simulink model "AGMD_model_R2024b"  (R2024b)
settings: Solver=VariableStepAuto  StartTime=0.0  StopTime=10.0  RelTol=1e-3
settings Model: Creator=Jan.Seemann  LastModifiedBy=Jan.Seemann

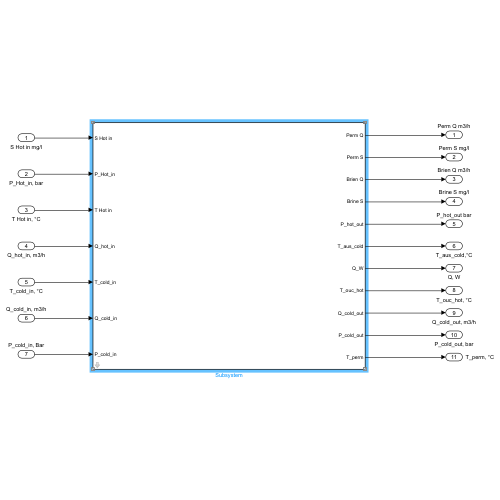
[thumbnail: Simulink's stored preview of the top-level diagram]
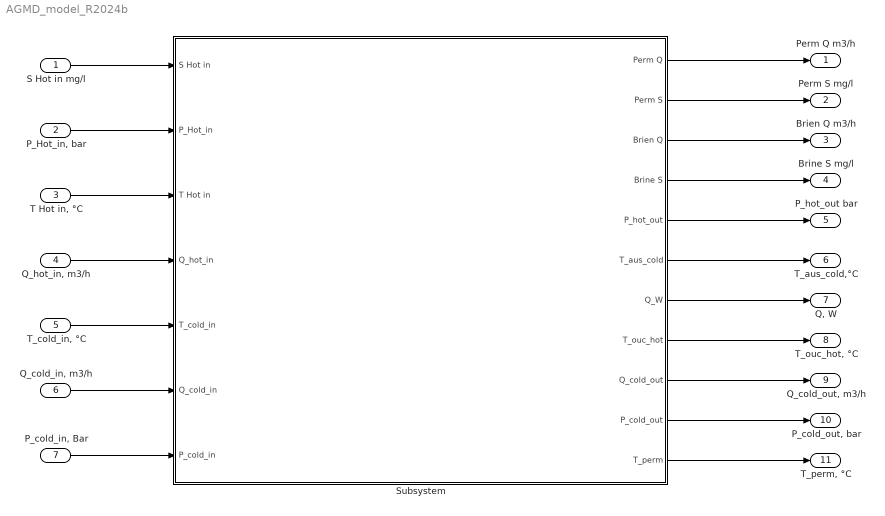
== system AGMD_model_R2024b ==
  S Hot in mg/l : Inport
  "P_Hot_in, bar" : Inport  Port=2
  "T Hot in, °C" : Inport  Port=3
  "Q_hot_in, m3/h" : Inport  Port=4
  "T_cold_in, °C" : Inport  Port=5
  "Q_cold_in, m3/h" : Inport  Port=6
  "P_cold_in, Bar" : Inport  Port=7
  Subsystem : Subsystem  mask{A=15, R=0.9999999, CCP=4000, HCP=4000, Dicke_Air=62/1000/1000, Dicke_cp=62/1000/1000, Dicke_M=69/1000/1000, K_air=0.0025, K_cp=0.5, K_m=0.25, DPCold=0, DPHOt=0, L=11.6}
      mask prompts: A "Area"; R "Recejectionratio"; CCP "heat capacity Cold Fluid, J/kgK"; HCP "heat capacity Hot Fluid, J/kgK"; Dicke_Air "Space Air, m"; Dicke_cp "thickness Cooling Platte, m"; Dicke_M "thickness Membrane, m"; K_air "Thermal conductivity Air, W/mK"; K_cp "Thermal conductivity Cooling Platte, W/mK"; K_m "Thermal conductivity Membrane, W/mK"; DPCold "Pressure drop ColdTube, bar"; DPHOt "Pressure drop Hot Tube, bar"; L "Chara. Length, m"
  Perm Q m3/h : Outport
  Perm S mg/l : Outport  Port=2
  Brien Q m3/h : Outport  Port=3
  Brine S mg/l : Outport  Port=4
  P_hot_out bar : Outport  Port=5
  T_aus_cold,°C : Outport  Port=6
  "Q, W" : Outport  Port=7
  "T_ouc_hot, °C" : Outport  Port=8
  "Q_cold_out, m3/h" : Outport  Port=9
  "P_cold_out, bar" : Outport  Port=10
  "T_perm, °C" : Outport  Port=11
  wires:
  Subsystem/1(Perm Q) -> Perm Q m3/h/1
  Subsystem/2(Perm S) -> Perm S mg/l/1
  Subsystem/3(Brien Q) -> Brien Q m3/h/1
  Subsystem/4(Brine S) -> Brine S mg/l/1
  Subsystem/5(P_hot_out) -> P_hot_out bar/1
  Subsystem/6(T_aus_cold) -> T_aus_cold,°C/1
  Subsystem/7(Q_W) -> "Q, W"/1
  Subsystem/8(T_ouc_hot) -> "T_ouc_hot, °C"/1
  Subsystem/9(Q_cold_out) -> "Q_cold_out, m3/h"/1
  Subsystem/10(P_cold_out) -> "P_cold_out, bar"/1
  Subsystem/11(T_perm) -> "T_perm, °C"/1
  S Hot in mg/l/1 -> Subsystem/1(S Hot in)
  "P_Hot_in, bar"/1 -> Subsystem/2(P_Hot_in)
  "T Hot in, °C"/1 -> Subsystem/3(T Hot in)
  "Q_hot_in, m3/h"/1 -> Subsystem/4(Q_hot_in)
  "T_cold_in, °C"/1 -> Subsystem/5(T_cold_in)
  "Q_cold_in, m3/h"/1 -> Subsystem/6(Q_cold_in)
  "P_cold_in, Bar"/1 -> Subsystem/7(P_cold_in)

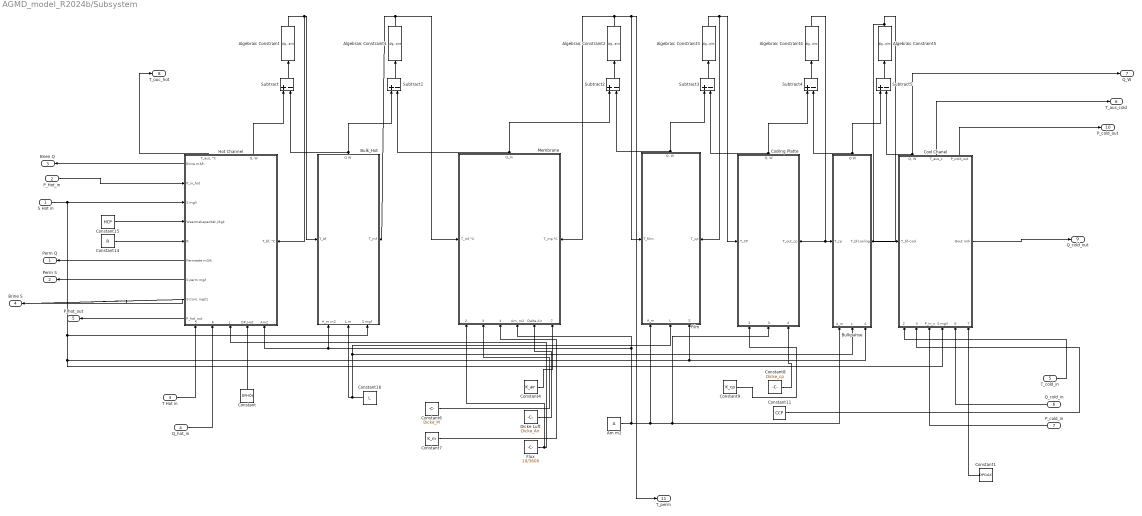
== system AGMD_model_R2024b/Subsystem ==
  S Hot in : Inport
  P_Hot_in : Inport  Port=2
  T Hot in : Inport  Port=3
  Q_hot_in : Inport  Port=4
  T_cold_in : Inport  Port=5
  Q_cold_in : Inport  Port=6
  P_cold_in : Inport  Port=7
  Algebraic Constraint{,1..5} (6 alike) : AlgebraicConstraint
  Am m2 : Constant  Value=A
  Bulk_Hot : Subsystem
      settings: PortSchema="{\"entries\":[{\"content\":{\"sides\":[{\"content\":{\"connectorIds\":[\"In1\"]},\"type\":\"ConnectorPlacement.EquallySpacedRectSide\",\"uuid\":\"ef4b2b41-cf19-4205-8bdd-c88c0c8e6088\"},{\"content\":{\"connectorIds\":[\"In5\"],\"side\":\"RIGHT\"},\"type\":\"ConnectorPlacement.EquallySpacedRectSide\",\"uuid\":\"90a0e595-a90d-4955-971b-cbb17d54f339\"},{\"content\":{\"connectorIds\":[\"Out1\"],\"side\":\"TOP\"},\"type\":\"ConnectorPlacement.EquallySpacedRectSide\",\"uuid\":\"ac71d737-c091-4b4d-923a-bfea117e1c9e\"},{\"content\":{\"connectorIds\":[\"In2\",\"In3\",\"In4\"],\"side\":\"BOTTOM\"},\"type\":\"ConnectorPlacement.EquallySpacedRectSide\",\"uuid\":\"c078efbb-00a2-4bad-921f-0a538f18104b\"}]},\"type\":\"ConnectorPlacement.EquallySpacedConnector\",\"uuid\":\"3aaa503e-a2b4-481c-8e52-42dcdd859844\"}],\"packageUris\":[\"http://schema.mathworks.com/mf0/Connector/R2020b\"],\"version\":\"1.0\"}"
  Bulkpahse : Subsystem
      settings: PortSchema="{\"entries\":[{\"content\":{\"sides\":[{\"content\":{\"connectorIds\":[\"In1\"]},\"type\":\"ConnectorPlacement.EquallySpacedRectSide\",\"uuid\":\"cd83c780-39a7-488d-a3d5-66e3425d7f86\"},{\"content\":{\"connectorIds\":[\"In5\"],\"side\":\"RIGHT\"},\"type\":\"ConnectorPlacement.EquallySpacedRectSide\",\"uuid\":\"ad4f5b7f-34f2-414c-8bc1-990d5ddf120f\"},{\"content\":{\"connectorIds\":[\"Out1\"],\"side\":\"TOP\"},\"type\":\"ConnectorPlacement.EquallySpacedRectSide\",\"uuid\":\"d94043ec-1d76-4835-9fe5-55fe607ca13f\"},{\"content\":{\"connectorIds\":[\"In2\",\"In3\",\"In4\"],\"side\":\"BOTTOM\"},\"type\":\"ConnectorPlacement.EquallySpacedRectSide\",\"uuid\":\"b1fdfa3b-d721-4849-9383-0fd7a2ff7ce1\"}]},\"type\":\"ConnectorPlacement.EquallySpacedConnector\",\"uuid\":\"49b2ce75-7c12-4465-a9d1-22146559eb16\"}],\"packageUris\":[\"http://schema.mathworks.com/mf0/Connector/R2020b\"],\"version\":\"1.0\"}"
  Constant : Constant  Value=DPHOt
  Constant1 : Constant  Value=DPCold
  Constant11 : Constant  Value=CCP
  Constant14 : Constant  Value=R
  Constant15 : Constant  Value=HCP
  Constant16 : Constant  Value=L
  Constant4 : Constant  Value=K_air
  Constant6 : Constant  Value=Dicke_M
  Constant7 : Constant  Value=K_m
  Constant8 : Constant  Value=Dicke_cp
  Constant9 : Constant  Value=K_cp
  Cool Chanel : Subsystem
      settings: PortSchema="{\"entries\":[{\"content\":{\"sides\":[{\"content\":{\"connectorIds\":[\"In1\"]},\"type\":\"ConnectorPlacement.EquallySpacedRectSide\",\"uuid\":\"c448acfc-f6aa-48b6-b853-5d81d9281dc0\"},{\"content\":{\"connectorIds\":[\"Out1\"],\"side\":\"RIGHT\"},\"type\":\"ConnectorPlacement.EquallySpacedRectSide\",\"uuid\":\"7e575c83-2c86-4510-ae36-745e6aa83247\"},{\"content\":{\"connectorIds\":[\"Out2\",\"Out3\",\"Out4\"],\"side\":\"TOP\"},\"type\":\"ConnectorPlacement.EquallySpacedRectSide\",\"uuid\":\"4a6df9d2-b5c9-43f7-a3d9-0ac9bbe4b67a\"},{\"content\":{\"connectorIds\":[\"In2\",\"In3\",\"In4\",\"In5\",\"In6\",\"In7\"],\"side\":\"BOTTOM\"},\"type\":\"ConnectorPlacement.EquallySpacedRectSide\",\"uuid\":\"eac96ba6-fa95-4e63-96f7-b902511d10a6\"}]},\"type\":\"ConnectorPlacement.EquallySpacedConnector\",\"uuid\":\"289f5ba6-df51-43a8-9e65-4dc3058f2d7c\"}],\"packageUris\":[\"http://schema.mathworks.com/mf0/Connector/R2020b\"],\"version\":\"1.0\"}"
  Cooling Platte : Subsystem
      settings: PortSchema="{\"entries\":[{\"content\":{\"sides\":[{\"content\":{\"connectorIds\":[\"In1\"]},\"type\":\"ConnectorPlacement.EquallySpacedRectSide\",\"uuid\":\"c07f3d14-23da-4d6c-a231-b487d35cf23a\"},{\"content\":{\"connectorIds\":[\"In5\"],\"side\":\"RIGHT\"},\"type\":\"ConnectorPlacement.EquallySpacedRectSide\",\"uuid\":\"132dff7f-1270-4e73-a49f-8e3c493cbf76\"},{\"content\":{\"connectorIds\":[\"Out1\"],\"side\":\"TOP\"},\"type\":\"ConnectorPlacement.EquallySpacedRectSide\",\"uuid\":\"f42b61b3-9665-4b68-99ce-b4151b983a04\"},{\"content\":{\"connectorIds\":[\"In2\",\"In3\",\"In4\"],\"side\":\"BOTTOM\"},\"type\":\"ConnectorPlacement.EquallySpacedRectSide\",\"uuid\":\"3d6787e6-2f20-4c5d-b35a-cc189669d767\"}]},\"type\":\"ConnectorPlacement.EquallySpacedConnector\",\"uuid\":\"48e32856-75ee-4ce0-8b78-4952240158a6\"}],\"packageUris\":[\"http://schema.mathworks.com/mf0/Connector/R2020b\"],\"version\":\"1.0\"}"
  "Dicke Luft " : Constant  Value=Dicke_Air
  Film : Subsystem
      settings: PortSchema="{\"entries\":[{\"content\":{\"sides\":[{\"content\":{\"connectorIds\":[\"In1\"]},\"type\":\"ConnectorPlacement.EquallySpacedRectSide\",\"uuid\":\"015337e1-8a5a-4833-8b0f-5ab9d6f3a80e\"},{\"content\":{\"connectorIds\":[\"In5\"],\"side\":\"RIGHT\"},\"type\":\"ConnectorPlacement.EquallySpacedRectSide\",\"uuid\":\"ffe29c11-abce-4f62-86d7-78803d541e75\"},{\"content\":{\"connectorIds\":[\"Out1\"],\"side\":\"TOP\"},\"type\":\"ConnectorPlacement.EquallySpacedRectSide\",\"uuid\":\"6e7e379e-b700-4f80-905d-b6d3887cb320\"},{\"content\":{\"connectorIds\":[\"In2\",\"In3\",\"In4\"],\"side\":\"BOTTOM\"},\"type\":\"ConnectorPlacement.EquallySpacedRectSide\",\"uuid\":\"39f7c5ec-6303-4d87-b419-58dfdd6ec091\"}]},\"type\":\"ConnectorPlacement.EquallySpacedConnector\",\"uuid\":\"e7928b9b-306f-421e-9818-1e4095991db6\"}],\"packageUris\":[\"http://schema.mathworks.com/mf0/Connector/R2020b\"],\"version\":\"1.0\"}"
  Flux : Constant  Value=10/3600
  Hot Channel : Subsystem
      settings: PortSchema="{\"entries\":[{\"content\":{\"sides\":[{\"content\":{\"connectorIds\":[\"Out3\",\"In1\",\"In2\",\"In3\",\"In4\",\"Out4\",\"Out5\",\"Out6\",\"Out7\"]},\"type\":\"ConnectorPlacement.EquallySpacedRectSide\",\"uuid\":\"fbc7a68d-5beb-43dd-a6f0-b755d0c17893\"},{\"content\":{\"connectorIds\":[\"In10\"],\"side\":\"RIGHT\"},\"type\":\"ConnectorPlacement.EquallySpacedRectSide\",\"uuid\":\"0716d393-5c1b-482d-88d7-1d54bbed30c8\"},{\"content\":{\"connectorIds\":[\"Out1\",\"Out2\"],\"side\":\"TOP\"},\"type\":\"ConnectorPlacement.EquallySpacedRectSide\",\"uuid\":\"7cadc919-8496-492b-8ec9-a6875040d21a\"},{\"content\":{\"connectorIds\":[\"In5\",\"In6\",\"In7\",\"In8\",\"In9\"],\"side\":\"BOTTOM\"},\"type\":\"ConnectorPlacement.EquallySpacedRectSide\",\"uuid\":\"ee11a940-0fee-47a3-9594-370a89fbc708\"}]},\"type\":\"ConnectorPlacement.EquallySpacedConnector\",\"uuid\":\"ba3bcdcd-a15a-4c6e-8936-726ab8cfa6f6\"}],\"packageUris\":[\"http://schema.mathworks.com/mf0/Connector/R2020b\"],\"version\":\"1.0\"}"
  Membrane : Subsystem
      settings: PortSchema="{\"entries\":[{\"content\":{\"sides\":[{\"content\":{\"connectorIds\":[\"In1\"]},\"type\":\"ConnectorPlacement.EquallySpacedRectSide\",\"uuid\":\"cd69aa9c-a695-4ae3-919f-da2064161930\"},{\"content\":{\"connectorIds\":[\"In8\"],\"side\":\"RIGHT\"},\"type\":\"ConnectorPlacement.EquallySpacedRectSide\",\"uuid\":\"a625c06c-887d-4646-98b1-3b4393effb73\"},{\"content\":{\"connectorIds\":[\"Out1\"],\"side\":\"TOP\"},\"type\":\"ConnectorPlacement.EquallySpacedRectSide\",\"uuid\":\"4b547f2f-723c-4068-9bd6-c942a8ec2112\"},{\"content\":{\"connectorIds\":[\"In2\",\"In3\",\"In4\",\"In5\",\"In6\",\"In7\"],\"side\":\"BOTTOM\"},\"type\":\"ConnectorPlacement.EquallySpacedRectSide\",\"uuid\":\"bf68c9ad-e157-4c0d-9a2b-c7fd1689a3f4\"}]},\"type\":\"ConnectorPlacement.EquallySpacedConnector\",\"uuid\":\"d2d78d85-b2cf-48d3-9a1a-b69a88097481\"}],\"packageUris\":[\"http://schema.mathworks.com/mf0/Connector/R2020b\"],\"version\":\"1.0\"}"
  Subtract{,1..5} (6 alike) : Sum  Inputs=+-
  Perm Q : Outport
  Perm S : Outport  Port=2
  Brien Q : Outport  Port=3
  Brine S : Outport  Port=4
  P_hot_out : Outport  Port=5
  T_aus_cold : Outport  Port=6
  Q_W : Outport  Port=7
  T_ouc_hot : Outport  Port=8
  Q_cold_out : Outport  Port=9
  P_cold_out : Outport  Port=10
  T_perm : Outport  Port=11
  wires:
  Algebraic Constraint1/1 -> Membrane/1(T_mf,°C), Bulk_Hot/5(T_mf)
  Q_hot_in/1 -> Hot Channel/6(Q Hot m3/h)
  Hot Channel/5(S perm mg/l) -> Perm S/1
  Constant8/1 -> Cooling Platte/4(Delta Paltte Cooling)
  Cool Chanel/3(T_aus_c) -> T_aus_cold/1
  Membrane/1(Q_m) -> Subtract1/2, Subtract2/1
  Constant9/1 -> Cooling Platte/2(Waermeleitfaehigkeit Platte)
  Subtract5/1 -> Algebraic Constraint5/1
  Bulk_Hot/1(Q W) -> Subtract/2, Subtract1/1
  Cool Chanel/4(P_cold_out) -> P_cold_out/1
  Am m2/1 -> Bulkpahse/2(A_m), Cooling Platte/3(Flaeche der Cooling Platte), Film/2(A_m), Hot Channel/9(Am2), Bulk_Hot/2(A_m m2), Membrane/5("Am, m2")
  Constant11/1 -> Cool Chanel/3(Waermekapazität J/kgK)
  Subtract1/1 -> Algebraic Constraint1/1
  Cool Chanel/1(Qout m/h) -> Q_cold_out/1
  S Hot in/1 -> Bulkpahse/4(S), Film/4(S), Cool Chanel/5(S mg/l), Bulk_Hot/4(S mg/l), Hot Channel/2(S mg/l)
  Algebraic Constraint4/1 -> Cooling Platte/5(T_out_cp), Bulkpahse/1(T_cp)
  Subtract/1 -> Algebraic Constraint/1
  Algebraic Constraint5/1 -> Cool Chanel/1(T_bf-cool), Bulkpahse/5(T_bfcooling)
  P_cold_in/1 -> Cool Chanel/4(P_in_c)
  "Dicke Luft "/1 -> Membrane/6(Dalta Air)
  T_cold_in/1 -> Cool Chanel/2(T_cooling_ein)
  P_Hot_in/1 -> Hot Channel/1(P_in_hot)
  Cool Chanel/2("Q, W") -> Q_W/1, Subtract5/2
  Constant16/1 -> Bulkpahse/3(L), Film/3(L), Bulk_Hot/3(L m)
  Hot Channel/1("T_aus, °C") -> T_ouc_hot/1
  Bulkpahse/1(Q W) -> Subtract5/1, Subtract4/2
  Hot Channel/7(P_hot_out) -> P_hot_out/1
  Hot Channel/6(S Conc mg/l1) -> Brine S/1
  Flux/1 -> Hot Channel/7(J), Membrane/2("J, kg/sm2")
  Constant14/1 -> Hot Channel/4(R)
  Film/1("Q, W") -> Subtract2/2, Subtract3/1
  Subtract3/1 -> Algebraic Constraint3/1
  T Hot in/1 -> Hot Channel/5("T_h_ein, °C")
  Q_cold_in/1 -> Cool Chanel/6(Q cold m3/h)
  Constant4/1 -> Membrane/7("k_air, W/mK")
  Hot Channel/3(Brine m3/h) -> Brien Q/1
  Constant1/1 -> Cool Chanel/7(DPCOld)
  Algebraic Constraint3/1 -> Cooling Platte/1(T_CP), Film/5(T_cp)
  Constant15/1 -> Hot Channel/3(Waermekapazität j/kgk)
  Algebraic Constraint2/1 -> T_perm/1, Film/1(T_film), Membrane/8(T_mp,°C)
  Subtract4/1 -> Algebraic Constraint4/1
  Constant7/1 -> Membrane/4("k_m, W/mK")
  Constant6/1 -> Membrane/3("delta_m, m")
  Hot Channel/4(Permeate m3/h) -> Perm Q/1
  Constant/1 -> Hot Channel/8(DP_Hot)
  Cooling Platte/1("Q, W") -> Subtract3/2, Subtract4/1
  Algebraic Constraint/1 -> Hot Channel/10("T_bf, °C"), Bulk_Hot/1(T_bf)
  Hot Channel/2("Q, W") -> Subtract/1
  Subtract2/1 -> Algebraic Constraint2/1

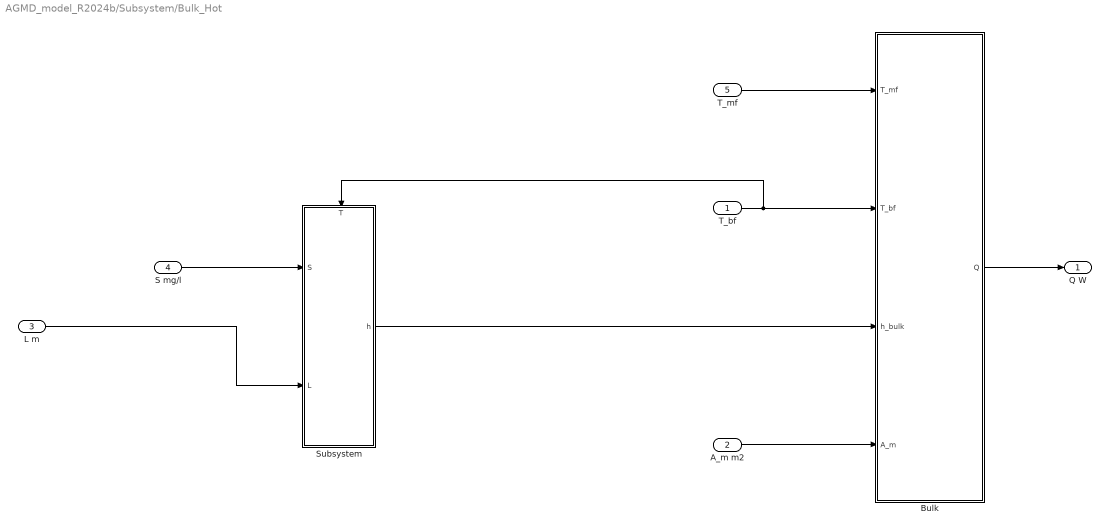
== system AGMD_model_R2024b/Subsystem/Bulk_Hot ==
  T_bf : Inport
  A_m m2 : Inport  Port=2
  L m : Inport  Port=3
  S mg/l : Inport  Port=4
  T_mf : Inport  Port=5
  Bulk : MATLAB Function  TreatAsAtomicUnit=on
  Subsystem : Subsystem
      settings: PortSchema="{\"entries\":[{\"content\":{\"sides\":[{\"content\":{\"connectorIds\":[\"In1\",\"In2\"]},\"type\":\"ConnectorPlacement.EquallySpacedRectSide\",\"uuid\":\"4135ebe6-441f-43d7-9be9-d9525d176f2c\"},{\"content\":{\"connectorIds\":[\"Out1\"],\"side\":\"RIGHT\"},\"type\":\"ConnectorPlacement.EquallySpacedRectSide\",\"uuid\":\"d9e7871b-5841-4db7-96fe-8558ee3ebd7a\"},{\"content\":{\"connectorIds\":[\"In3\"],\"side\":\"TOP\"},\"type\":\"ConnectorPlacement.EquallySpacedRectSide\",\"uuid\":\"bca1fa39-ae4b-46e6-af8d-7fe20692a0ee\"}]},\"type\":\"ConnectorPlacement.EquallySpacedConnector\",\"uuid\":\"33afa6da-10b0-4c15-8b5e-951d2ae663b7\"}],\"packageUris\":[\"http://schema.mathworks.com/mf0/Connector/R2020b\"],\"version\":\"1.0\"}"
  Q W : Outport
  wires:
  Bulk/1(Q) -> Q W/1
  T_mf/1 -> Bulk/1(T_mf)
  T_bf/1 -> Bulk/2(T_bf), Subsystem/3(T)
  A_m m2/1 -> Bulk/4(A_m)
  S mg/l/1 -> Subsystem/1(S)
  L m/1 -> Subsystem/2(L)
  Subsystem/1(h) -> Bulk/3(h_bulk)

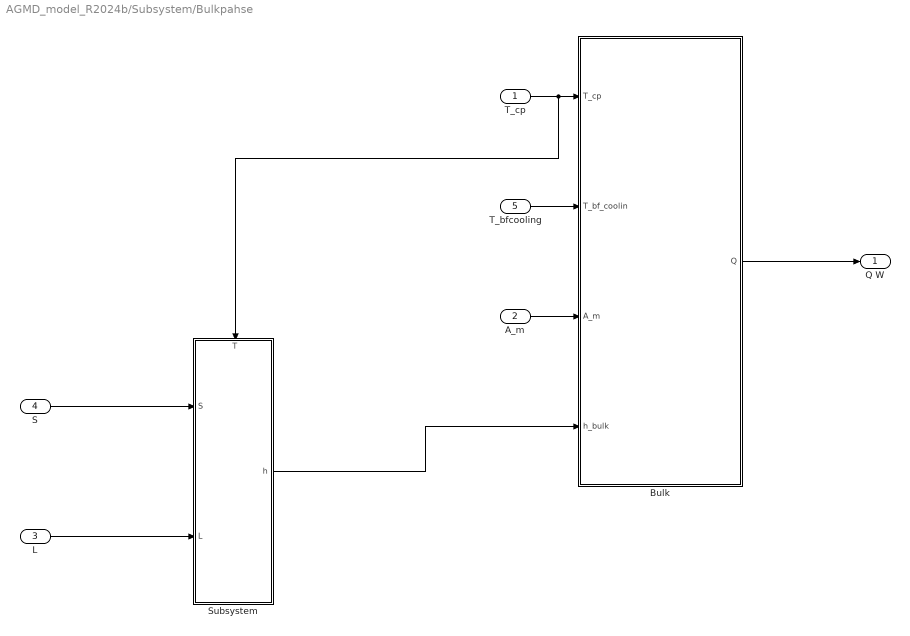
== system AGMD_model_R2024b/Subsystem/Bulkpahse ==
  T_cp : Inport
  A_m : Inport  Port=2
  L : Inport  Port=3
  S : Inport  Port=4
  T_bfcooling : Inport  Port=5
  Bulk : MATLAB Function  TreatAsAtomicUnit=on
  Subsystem : Subsystem
      settings: PortSchema="{\"entries\":[{\"content\":{\"sides\":[{\"content\":{\"connectorIds\":[\"In1\",\"In2\"]},\"type\":\"ConnectorPlacement.EquallySpacedRectSide\",\"uuid\":\"4135ebe6-441f-43d7-9be9-d9525d176f2c\"},{\"content\":{\"connectorIds\":[\"Out1\"],\"side\":\"RIGHT\"},\"type\":\"ConnectorPlacement.EquallySpacedRectSide\",\"uuid\":\"d9e7871b-5841-4db7-96fe-8558ee3ebd7a\"},{\"content\":{\"connectorIds\":[\"In3\"],\"side\":\"TOP\"},\"type\":\"ConnectorPlacement.EquallySpacedRectSide\",\"uuid\":\"bca1fa39-ae4b-46e6-af8d-7fe20692a0ee\"}]},\"type\":\"ConnectorPlacement.EquallySpacedConnector\",\"uuid\":\"33afa6da-10b0-4c15-8b5e-951d2ae663b7\"}],\"packageUris\":[\"http://schema.mathworks.com/mf0/Connector/R2020b\"],\"version\":\"1.0\"}"
  Q W : Outport
  wires:
  Bulk/1(Q) -> Q W/1
  T_cp/1 -> Subsystem/3(T), Bulk/1(T_cp)
  T_bfcooling/1 -> Bulk/2(T_bf_coolin)
  A_m/1 -> Bulk/3(A_m)
  S/1 -> Subsystem/1(S)
  L/1 -> Subsystem/2(L)
  Subsystem/1(h) -> Bulk/4(h_bulk)

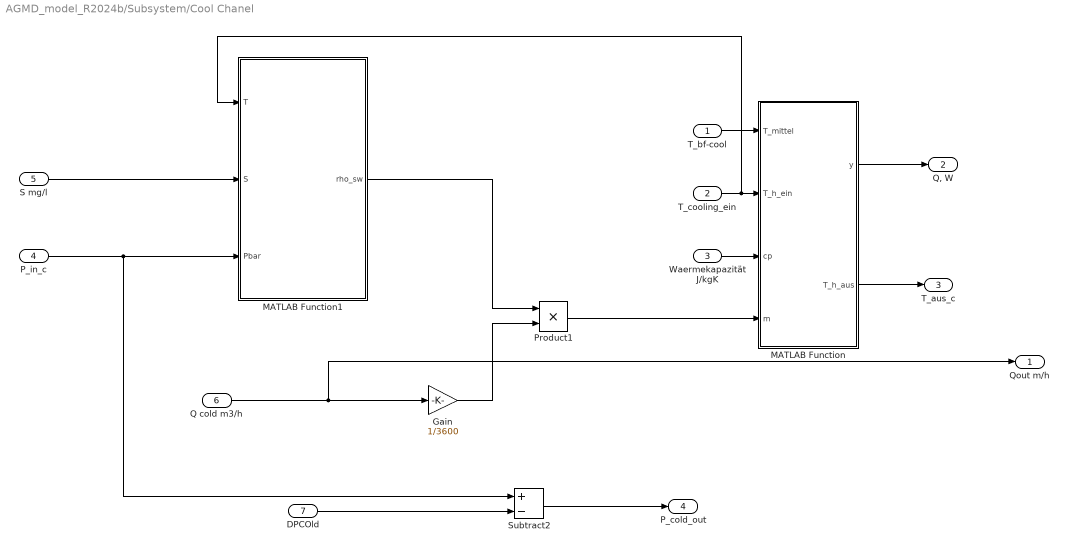
== system AGMD_model_R2024b/Subsystem/Cool Chanel ==
  T_bf-cool : Inport
  T_cooling_ein : Inport  Port=2
  Waermekapazität J/kgK : Inport  Port=3
  P_in_c : Inport  Port=4
  S mg/l : Inport  Port=5
  Q cold m3/h : Inport  Port=6
  DPCOld : Inport  Port=7
  Gain : Gain  Gain=1/3600
  MATLAB Function : MATLAB Function  TreatAsAtomicUnit=on
  MATLAB Function1 : MATLAB Function  TreatAsAtomicUnit=on
  Product1 : Product
  Subtract2 : Sum  Inputs=+-
  Qout m/h : Outport
  "Q, W" : Outport  Port=2
  T_aus_c : Outport  Port=3
  P_cold_out : Outport  Port=4
  wires:
  MATLAB Function/2(T_h_aus) -> T_aus_c/1
  MATLAB Function/1(y) -> "Q, W"/1
  T_bf-cool/1 -> MATLAB Function/1(T_mittel)
  Waermekapazität J/kgK/1 -> MATLAB Function/3(cp)
  MATLAB Function1/1(rho_sw) -> Product1/1
  T_cooling_ein/1 -> MATLAB Function1/1(T), MATLAB Function/2(T_h_ein)
  S mg/l/1 -> MATLAB Function1/2(S)
  Q cold m3/h/1 -> Qout m/h/1, Gain/1
  Gain/1 -> Product1/2
  P_in_c/1 -> Subtract2/1, MATLAB Function1/3(Pbar)
  Product1/1 -> MATLAB Function/4(m)
  Subtract2/1 -> P_cold_out/1
  DPCOld/1 -> Subtract2/2

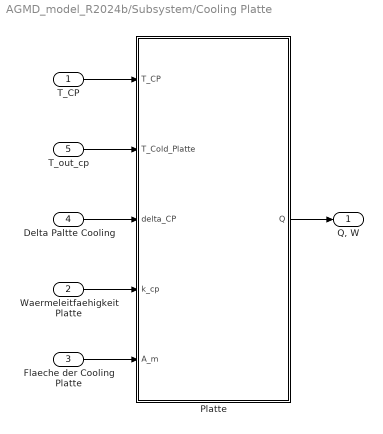
== system AGMD_model_R2024b/Subsystem/Cooling Platte ==
  T_CP : Inport
  Waermeleitfaehigkeit Platte : Inport  Port=2
  Flaeche der Cooling Platte : Inport  Port=3
  Delta Paltte Cooling : Inport  Port=4
  T_out_cp : Inport  Port=5
  Platte : MATLAB Function  TreatAsAtomicUnit=on
  "Q, W" : Outport
  wires:
  T_out_cp/1 -> Platte/2(T_Cold_Platte)
  T_CP/1 -> Platte/1(T_CP)
  Delta Paltte Cooling/1 -> Platte/3(delta_CP)
  Waermeleitfaehigkeit Platte/1 -> Platte/4(k_cp)
  Flaeche der Cooling Platte/1 -> Platte/5(A_m)
  Platte/1(Q) -> "Q, W"/1

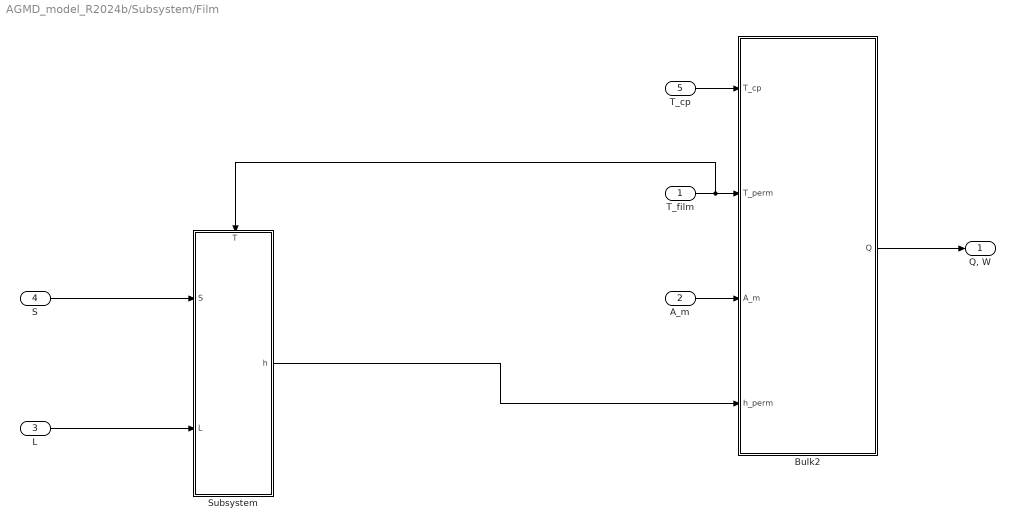
== system AGMD_model_R2024b/Subsystem/Film ==
  T_film : Inport
  A_m : Inport  Port=2
  L : Inport  Port=3
  S : Inport  Port=4
  T_cp : Inport  Port=5
  Bulk2 : MATLAB Function  TreatAsAtomicUnit=on
  Subsystem : Subsystem
      settings: PortSchema="{\"entries\":[{\"content\":{\"sides\":[{\"content\":{\"connectorIds\":[\"In1\",\"In2\"]},\"type\":\"ConnectorPlacement.EquallySpacedRectSide\",\"uuid\":\"4135ebe6-441f-43d7-9be9-d9525d176f2c\"},{\"content\":{\"connectorIds\":[\"Out1\"],\"side\":\"RIGHT\"},\"type\":\"ConnectorPlacement.EquallySpacedRectSide\",\"uuid\":\"d9e7871b-5841-4db7-96fe-8558ee3ebd7a\"},{\"content\":{\"connectorIds\":[\"In3\"],\"side\":\"TOP\"},\"type\":\"ConnectorPlacement.EquallySpacedRectSide\",\"uuid\":\"bca1fa39-ae4b-46e6-af8d-7fe20692a0ee\"}]},\"type\":\"ConnectorPlacement.EquallySpacedConnector\",\"uuid\":\"33afa6da-10b0-4c15-8b5e-951d2ae663b7\"}],\"packageUris\":[\"http://schema.mathworks.com/mf0/Connector/R2020b\"],\"version\":\"1.0\"}"
  "Q, W" : Outport
  wires:
  T_cp/1 -> Bulk2/1(T_cp)
  T_film/1 -> Subsystem/3(T), Bulk2/2(T_perm)
  Bulk2/1(Q) -> "Q, W"/1
  A_m/1 -> Bulk2/3(A_m)
  L/1 -> Subsystem/2(L)
  Subsystem/1(h) -> Bulk2/4(h_perm)
  S/1 -> Subsystem/1(S)

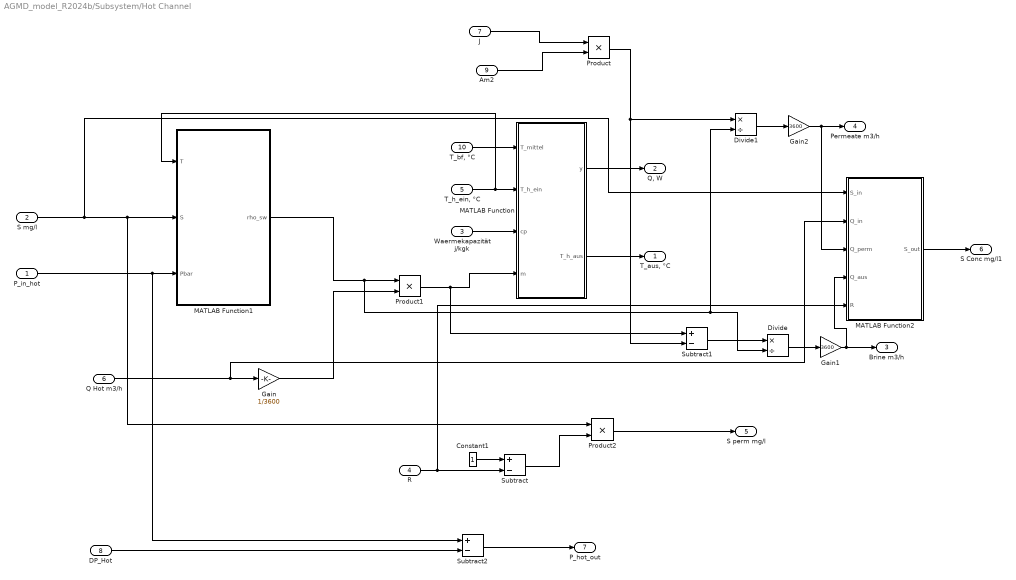
== system AGMD_model_R2024b/Subsystem/Hot Channel ==
  P_in_hot : Inport
  S mg/l : Inport  Port=2
  Waermekapazität j/kgk : Inport  Port=3
  R : Inport  Port=4
  "T_h_ein, °C" : Inport  Port=5
  Q Hot m3/h : Inport  Port=6
  J : Inport  Port=7
  DP_Hot : Inport  Port=8
  Am2 : Inport  Port=9
  "T_bf, °C" : Inport  Port=10
  Constant1 : Constant
  Divide : Product  Inputs=*/
  Divide1 : Product  Inputs=*/
  Gain : Gain  Gain=1/3600
  Gain1 : Gain  Gain=3600
  Gain2 : Gain  Gain=3600
  MATLAB Function : MATLAB Function  TreatAsAtomicUnit=on
  MATLAB Function1 : MATLAB Function  TreatAsAtomicUnit=on
  MATLAB Function2 : MATLAB Function  TreatAsAtomicUnit=on
  Product : Product
  Product1 : Product
  Product2 : Product
  Subtract : Sum  Inputs=+-
  Subtract1 : Sum  Inputs=+-
  Subtract2 : Sum  Inputs=+-
  "T_aus, °C" : Outport
  "Q, W" : Outport  Port=2
  Brine m3/h : Outport  Port=3
  Permeate m3/h : Outport  Port=4
  S perm mg/l : Outport  Port=5
  S Conc mg/l1 : Outport  Port=6
  P_hot_out : Outport  Port=7
  wires:
  J/1 -> Product/1
  MATLAB Function/1(y) -> "Q, W"/1
  "T_bf, °C"/1 -> MATLAB Function/1(T_mittel)
  Waermekapazität j/kgk/1 -> MATLAB Function/3(cp)
  MATLAB Function/2(T_h_aus) -> "T_aus, °C"/1
  "T_h_ein, °C"/1 -> MATLAB Function1/1(T), MATLAB Function/2(T_h_ein)
  R/1 -> MATLAB Function2/5(R), Subtract/2
  Constant1/1 -> Subtract/1
  Am2/1 -> Product/2
  Product/1 -> Divide1/1, Subtract1/2
  P_in_hot/1 -> Subtract2/1, MATLAB Function1/3(Pbar)
  S mg/l/1 -> MATLAB Function2/1(S_in), Product2/1, MATLAB Function1/2(S)
  Q Hot m3/h/1 -> MATLAB Function2/2(Q_in), Gain/1
  MATLAB Function1/1(rho_sw) -> Divide1/2, Divide/2, Product1/1
  Product1/1 -> Subtract1/1, MATLAB Function/4(m)
  Gain/1 -> Product1/2
  Subtract1/1 -> Divide/1
  Divide/1 -> Gain1/1
  Gain2/1 -> MATLAB Function2/3(Q_perm), Permeate m3/h/1
  Divide1/1 -> Gain2/1
  Subtract/1 -> Product2/2
  Product2/1 -> S perm mg/l/1
  MATLAB Function2/1(S_out) -> S Conc mg/l1/1
  Gain1/1 -> MATLAB Function2/4(Q_aus), Brine m3/h/1
  DP_Hot/1 -> Subtract2/2
  Subtract2/1 -> P_hot_out/1

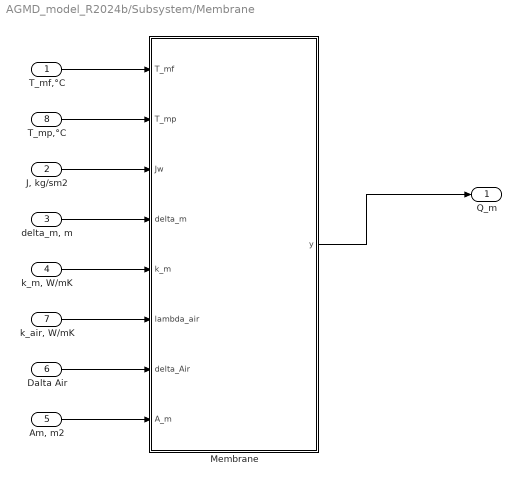
== system AGMD_model_R2024b/Subsystem/Membrane ==
  T_mf,°C : Inport
  "J, kg/sm2" : Inport  Port=2
  "delta_m, m" : Inport  Port=3
  "k_m, W/mK" : Inport  Port=4
  "Am, m2" : Inport  Port=5
  Dalta Air : Inport  Port=6
  "k_air, W/mK" : Inport  Port=7
  T_mp,°C : Inport  Port=8
  Membrane : MATLAB Function  TreatAsAtomicUnit=on
  Q_m : Outport
  wires:
  "J, kg/sm2"/1 -> Membrane/3(Jw)
  "delta_m, m"/1 -> Membrane/4(delta_m)
  "k_m, W/mK"/1 -> Membrane/5(k_m)
  "Am, m2"/1 -> Membrane/8(A_m)
  T_mf,°C/1 -> Membrane/1(T_mf)
  Membrane/1(y) -> Q_m/1
  T_mp,°C/1 -> Membrane/2(T_mp)
  "k_air, W/mK"/1 -> Membrane/6(lambda_air)
  Dalta Air/1 -> Membrane/7(delta_Air)

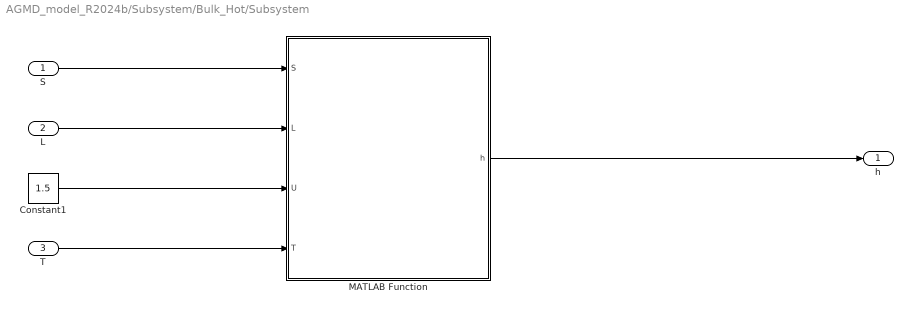
== system AGMD_model_R2024b/Subsystem/Bulk_Hot/Subsystem ==
  S : Inport
  L : Inport  Port=2
  T : Inport  Port=3
  Constant1 : Constant  Value=1.5
  MATLAB Function : MATLAB Function  TreatAsAtomicUnit=on
  h : Outport
  wires:
  L/1 -> MATLAB Function/2(L)
  MATLAB Function/1(h) -> h/1
  S/1 -> MATLAB Function/1(S)
  Constant1/1 -> MATLAB Function/3(U)
  T/1 -> MATLAB Function/4(T)

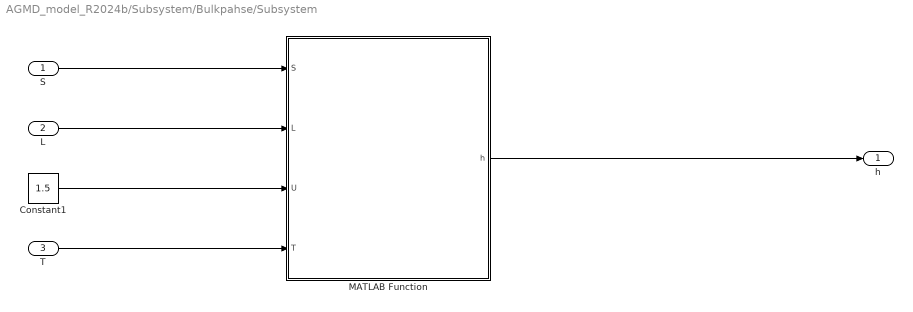
== system AGMD_model_R2024b/Subsystem/Bulkpahse/Subsystem ==
  S : Inport
  L : Inport  Port=2
  T : Inport  Port=3
  Constant1 : Constant  Value=1.5
  MATLAB Function : MATLAB Function  TreatAsAtomicUnit=on
  h : Outport
  wires:
  L/1 -> MATLAB Function/2(L)
  MATLAB Function/1(h) -> h/1
  S/1 -> MATLAB Function/1(S)
  Constant1/1 -> MATLAB Function/3(U)
  T/1 -> MATLAB Function/4(T)

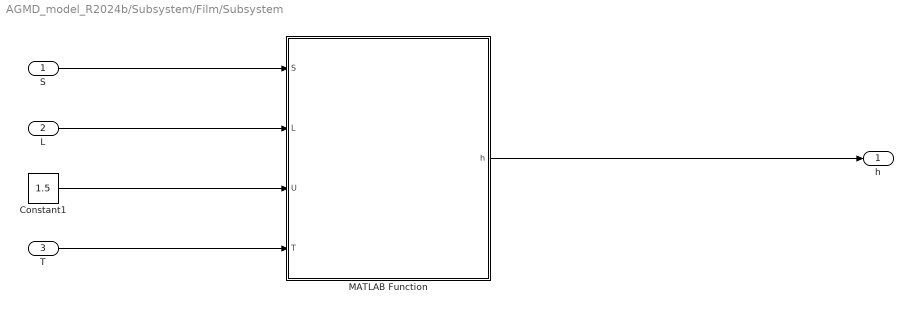
== system AGMD_model_R2024b/Subsystem/Film/Subsystem ==
  S : Inport
  L : Inport  Port=2
  T : Inport  Port=3
  Constant1 : Constant  Value=1.5
  MATLAB Function : MATLAB Function  TreatAsAtomicUnit=on
  h : Outport
  wires:
  L/1 -> MATLAB Function/2(L)
  MATLAB Function/1(h) -> h/1
  S/1 -> MATLAB Function/1(S)
  Constant1/1 -> MATLAB Function/3(U)
  T/1 -> MATLAB Function/4(T)

== matlab function AGMD_model_R2024b/Subsystem/Film/Bulk2 ==
  data: T_cp input; T_perm input; A_m input; Q output; h_perm input
function Q = fcn(T_cp,T_perm,A_m, h_perm)
% Determination of heat flow
Q = A_m * h_perm * (T_perm -T_cp ) ;

== matlab function AGMD_model_R2024b/Subsystem/Cooling Platte/Platte ==
  data: T_CP input; T_Cold_Platte input; Q output; delta_CP input; k_cp input; A_m input
function Q = fcn(T_CP, T_Cold_Platte , delta_CP,k_cp,A_m)
% Membrangeometrie
% A_m = 1.6;              % Membranfläche [m^2]
% delta_cp = 1.5e-3;      % Kühlplattenstärke [m]

% Wärmeleitfähigkeiten
% k_cp = 60;              % Kühlplatte [W/mK]

% Mittlere Temperatur in °K
T_mitte = (T_Cold_Platte + T_CP)/2 + 273.15;
% Verdampfungsentalpie in kJ/kg 
Hw = 1.75535 * T_mitte + 2024.3;
% Bestimmung der Wärmemengen
Q =  k_cp/delta_CP *(T_CP - T_Cold_Platte);

== matlab function AGMD_model_R2024b/Subsystem/Cool Chanel/MATLAB Function ==
  data: T_mittel input; y output; T_h_ein input; cp input; m input; T_h_aus output
function [y ,T_h_aus] = fcn(T_mittel, T_h_ein,cp,m)
% Bestimmungen der Ausgehenden Temperature mittels der Bulk Temperatur °C
T_h_aus = T_mittel*2 - T_h_ein;
% Bestimmung der Wärmemenge in W
y = cp * m * (T_h_aus - T_h_ein); % W

== matlab function AGMD_model_R2024b/Subsystem/Hot Channel/MATLAB Function2 ==
  data: S_in input; S_out output; Q_in input; Q_perm input; Q_aus input; R input
function S_out = fcn(S_in,Q_in,Q_perm,Q_aus,R)
% Mittels Komponenten bilanz bestimmung des aus Gehenden Salzgehaltes
% Determination of the salt content of the effluent using component balance
S_out = S_in *(Q_in - Q_perm*(1-R))/Q_aus;

== matlab function AGMD_model_R2024b/Subsystem/Bulk_Hot/Bulk ==
  data: T_mf input; Q output; T_bf input; h_bulk input; A_m input
function Q = fcn(T_mf, T_bf, h_bulk, A_m)
% Membrangeometrie
% A_m = 1.6;               % Membranearea [m^2]
% H_bulk = 2000;           % Wärmeübergangskoeffizient [W/Km²] / heat transfer coefficient
Q = A_m * h_bulk * (T_bf - T_mf) ; %W

== matlab function AGMD_model_R2024b/Subsystem/Membrane/Membrane ==
  data: T_mf input; y output; T_mp input; Jw input; delta_m input; k_m input; lambda_air input; delta_Air input; A_m input
function y = fcn(T_mf, T_mp, Jw , delta_m,k_m,lambda_air, delta_Air,A_m )
% Bildung der T_mittel Temperatur / Formation of the T_middle temperature
T_mitte = (T_mf + T_mp)/2 + 273.15;
% Bestimmung der Verdampfungsentlapie J/kg / Determination of evaporation enthalpy J/kg
% Quelle: http://dx.doi.org/10.1016/j.desal.2015.08.016
Hw = (1.75535 * T_mitte + 2024.3);

h = (delta_Air / lambda_air +delta_m /k_m + 1/7.3)^(-1);
% Bestimmung der Wärmestrom / Determination of heat flow
y =  k_m/delta_m *(T_mf -T_mp) * A_m +  Jw * A_m * Hw;

== matlab function AGMD_model_R2024b/Subsystem/Bulkpahse/Bulk ==
  data: T_cp input; Q output; T_bf_coolin input; A_m input; h_bulk input
function Q = fcn(T_cp , T_bf_coolin,A_m, h_bulk)
% Membrangeometrie
% A_m = 1.6;               % Membranfläche [m^2]
% H_bulk = 2000;           % Wärmeübergangskoeffizient [W/Km²] 



Q = A_m * h_bulk * (T_cp-T_bf_coolin) ; %m2 * w/m2K *K

== matlab function AGMD_model_R2024b/Subsystem/Bulk_Hot/Subsystem/MATLAB Function ==
  data: S input; L input; U input; T input; h output
function h = h_plate_meerwasser( S, L, U, T)
% Berechnet den Wärmeübergangskoeffizienten h [W/m^2K]
% für Meerwasser an einer ebenen Platte bei paralleler Umströmung
%
% Eingabeparameter:
% T  - Temperatur in °C
% S  - Salzgehalt in g/kg
% L  - charakteristische Länge der Platte in m
% U  - Strömungsgeschwindigkeit in m/s
%
% Ausgabe:
% h  - Wärmeübergangskoeffizient in W/m²K

% Calculates the heat transfer coefficient h [W/m^2K]
% for seawater on a flat plate with parallel flow
%
% Input parameters:
% T  - Temperature in °C
% S  - Salinity in g/kg
% L  - Characteristic length of the plate in m
% U  - Flow velocity in m/s
%
% Output:
% h  - Heat transfer coefficient in W/m²K

if T > 120
    T = 60;
end
S = S /1000; % von mg/l in g/kg

% --- Schritt 1: Materialeigenschaften für Meerwasser ---
% Näherungsweise: empirische Gleichungen aus Sharqawy et al. (Desalination, 2010)
% --- Step 1: Material properties for seawater ---
% Approximate: empirical equations from Sharqawy et al. (Desalination, 2010)
rho = 1000 -0.07*S + 0.2*T;         % Dichte [kg/m³]
mu = (1e-3)*(1 + 0.02*S/35 - 0.033*T/25);  % Viskosität [Pa·s] vereinfacht
cp = 4180 - 10*S;                    % Wärmekapazität [J/kg·K]
k = 0.6 - 0.001*T;                   % Wärmeleitfähigkeit [W/m·K]

% --- Schritt 2: Kenngrößen ---
nu = mu / rho;                      % Kinematische Viskosität [m²/s]
alpha = k / (rho * cp);            % Temperaturleitfähigkeit [m²/s]
Pr = nu / alpha;                   % Prandtl-Zahl
Re = U * L / nu;                   % Reynolds-Zahl

% --- Schritt 3: Nusselt-Zahl berechnen ---
if Re < 5e5
    Nu = 0.664 * Re^0.5 * Pr^(1/3);    % laminare Strömung (mittlerer Nu)
else
    Nu = 0.037 * Re^0.8 * Pr^(1/3);    % turbulente Strömung
end

% --- Schritt 4: Wärmeübergangskoeffizient ---
h = Nu * k / L;                      % [W/m²K]
end

== matlab function AGMD_model_R2024b/Subsystem/Hot Channel/MATLAB Function1 ==
  data: T input; rho_sw output; S input; Pbar input
function rho_sw = seawater_density(T, S, Pbar)
% Berechnet die Dichte von Meerwasser [kg/m³] für gegebene Temperatur T [°C], 
% Salzgehalt S [mg/kg] und Druck P [Pa]
% Basierend auf Sharqawy et al. (2010), Gleichungen (18)-(20)

    % Umrechnungen
    S_kgkg = S / 1000 /1000;      % Umwandlung in kg/kg
    P0 = 1e5;               % Atmosphärendruck [Pa]
    P = Pbar * 1e5; 

    % --- Koeffizienten (Gleichung 19) ---
    a1 = 9.999e2;
    a2 = 2.034e-2;
    a3 = -6.162e-3;
    a4 = 2.261e-5;
    a5 = -4.657e-8;

    b1 = 8.020e2;
    b2 = -2.001;
    b3 = 1.677e-2;
    b4 = -3.060e-5;
    b5 = -1.613e-5;

    % --- Koeffizienten (Gleichung 20) ---
    c1 = 5.0792e-4;
    c2 = -3.4168e-6;
    c3 = 5.6931e-10;
    c4 = -3.7263e-10;
    c5 = 1.4465e-12;
    c6 = -1.7058e-15;
    c7 = -1.3389e-6;
    c8 = 4.8603e-9;
    c9 = -6.8039e-10;

    d1 = -1.1077e-6;
    d2 = 5.5584e-9;
    d3 = -4.2539e-11;
    d4 = 8.3702e-9;

    % --- Temperaturabhängiger Basis-Term ρ(t,S,P0) ---
    rho_0 = (a1 + a2*T + a3*T.^2 + a4*T.^3 + a5*T.^4) + ...
            S_kgkg.*(b1 + b2*T + b3*T.^2 + b4*T.^3 + b5*T.^2);

    % --- Kompressionsfaktor F_P ---
    dP = P - P0;
    dP2 = (P.^2 - P0.^2)/2;

    term1 = dP .* (c1 + c2*T + c3*T.^2 + c4*T.^3 + c5*T.^4 + c6*T.^5 + ...
                   S.*(d1 + d2*T + d3*T.^2));
    term2 = dP2 .* (c7 + c8*T + c9*T.^3 + d4*S);

    F_P = exp(term1 + term2);

    % --- Gesamtdichte ---
    rho_sw = rho_0 .* F_P;
end

== matlab function AGMD_model_R2024b/Subsystem/Bulkpahse/Subsystem/MATLAB Function ==
  data: S input; L input; U input; T input; h output
function h = h_plate_meerwasser( S, L, U, T)
% Berechnet den Wärmeübergangskoeffizienten h [W/m^2K]
% für Meerwasser an einer ebenen Platte bei paralleler Umströmung
%
% Eingabeparameter:
% T  - Temperatur in °C
% S  - Salzgehalt in g/kg
% L  - charakteristische Länge der Platte in m
% U  - Strömungsgeschwindigkeit in m/s
%
% Ausgabe:
% h  - Wärmeübergangskoeffizient in W/m²K
if T > 120
    T = 60;
end
S = S /1000; % von mg/l in g/kg

% --- Schritt 1: Materialeigenschaften für Meerwasser ---
% Näherungsweise: empirische Gleichungen aus Sharqawy et al. (Desalination, 2010)

rho = 1000 -0.07*S + 0.2*T;         % Dichte [kg/m³]
mu = (1e-3)*(1 + 0.02*S/35 - 0.033*T/25);  % Viskosität [Pa·s] vereinfacht
cp = 4180 - 10*S;                    % Wärmekapazität [J/kg·K]
k = 0.6 - 0.001*T;                   % Wärmeleitfähigkeit [W/m·K]

% --- Schritt 2: Kenngrößen ---
nu = mu / rho;                      % Kinematische Viskosität [m²/s]
alpha = k / (rho * cp);            % Temperaturleitfähigkeit [m²/s]
Pr = nu / alpha;                   % Prandtl-Zahl
Re = U * L / nu;                   % Reynolds-Zahl

% --- Schritt 3: Nusselt-Zahl berechnen ---
if Re < 5e5
    Nu = 0.664 * Re^0.5 * Pr^(1/3);    % laminare Strömung (mittlerer Nu)
else
    Nu = 0.037 * Re^0.8 * Pr^(1/3);    % turbulente Strömung
end

% --- Schritt 4: Wärmeübergangskoeffizient ---
h = Nu * k / L;                      % [W/m²K]

end

== matlab function AGMD_model_R2024b/Subsystem/Film/Subsystem/MATLAB Function ==
  data: S input; L input; U input; T input; h output
function h = h_plate_meerwasser( S, L, U, T)
% Berechnet den Wärmeübergangskoeffizienten h [W/m^2K]
% für Meerwasser an einer ebenen Platte bei paralleler Umströmung
%
% Eingabeparameter:
% T  - Temperatur in °C
% S  - Salzgehalt in g/kg
% L  - charakteristische Länge der Platte in m
% U  - Strömungsgeschwindigkeit in m/s
%
% Ausgabe:
% h  - Wärmeübergangskoeffizient in W/m²K

% Calculates the heat transfer coefficient h [W/m^2K]
% for seawater on a flat plate with parallel flow
%
% Input parameters:
% T  - Temperature in °C
% S  - Salinity in g/kg
% L  - Characteristic length of the plate in m
% U  - Flow velocity in m/s
%
% Output:
% h  - Heat transfer coefficient in W/m²K

if T > 120
    T = 60;
end
S = S /1000; % von mg/l in g/kg

% --- Schritt 1: Materialeigenschaften für Meerwasser ---
% Näherungsweise: empirische Gleichungen aus Sharqawy et al. (Desalination, 2010)
% --- Step 1: Material properties for seawater ---
% Approximate: empirical equations from Sharqawy et al. (Desalination, 2010)
rho = 1000 -0.07*S + 0.2*T;         % Dichte [kg/m³]
mu = (1e-3)*(1 + 0.02*S/35 - 0.033*T/25);  % Viskosität [Pa·s] vereinfacht
cp = 4180 - 10*S;                    % Wärmekapazität [J/kg·K]
k = 0.6 - 0.001*T;                   % Wärmeleitfähigkeit [W/m·K]

% --- Schritt 2: Kenngrößen ---
nu = mu / rho;                      % Kinematische Viskosität [m²/s]
alpha = k / (rho * cp);            % Temperaturleitfähigkeit [m²/s]
Pr = nu / alpha;                   % Prandtl-Zahl
Re = U * L / nu;                   % Reynolds-Zahl

% --- Schritt 3: Nusselt-Zahl berechnen ---
if Re < 5e5
    Nu = 0.664 * Re^0.5 * Pr^(1/3);    % laminare Strömung (mittlerer Nu)
else
    Nu = 0.037 * Re^0.8 * Pr^(1/3);    % turbulente Strömung
end

% --- Schritt 4: Wärmeübergangskoeffizient ---
h = Nu * k / L;                      % [W/m²K]

end

== matlab function AGMD_model_R2024b/Subsystem/Cool Chanel/MATLAB Function1 ==
  data: T input; rho_sw output; S input; Pbar input
function rho_sw = seawater_density(T, S, Pbar)
% Berechnet die Dichte von Meerwasser [kg/m³] für gegebene Temperatur T [°C], 
% Salzgehalt S [mg/kg] und Druck P [Pa]
% Basierend auf Sharqawy et al. (2010), Gleichungen (18)-(20)

    % Umrechnungen
    S_kgkg = S / 1000 /1000;      % Umwandlung in kg/kg
    P0 = 1e5;               % Atmosphärendruck [Pa]
    P = Pbar * 1e5; 

    % --- Koeffizienten (Gleichung 19) ---
    a1 = 9.999e2;
    a2 = 2.034e-2;
    a3 = -6.162e-3;
    a4 = 2.261e-5;
    a5 = -4.657e-8;

    b1 = 8.020e2;
    b2 = -2.001;
    b3 = 1.677e-2;
    b4 = -3.060e-5;
    b5 = -1.613e-5;

    % --- Koeffizienten (Gleichung 20) ---
    c1 = 5.0792e-4;
    c2 = -3.4168e-6;
    c3 = 5.6931e-10;
    c4 = -3.7263e-10;
    c5 = 1.4465e-12;
    c6 = -1.7058e-15;
    c7 = -1.3389e-6;
    c8 = 4.8603e-9;
    c9 = -6.8039e-10;

    d1 = -1.1077e-6;
    d2 = 5.5584e-9;
    d3 = -4.2539e-11;
    d4 = 8.3702e-9;

    % --- Temperaturabhängiger Basis-Term ρ(t,S,P0) ---
    rho_0 = (a1 + a2*T + a3*T.^2 + a4*T.^3 + a5*T.^4) + ...
            S_kgkg.*(b1 + b2*T + b3*T.^2 + b4*T.^3 + b5*T.^2);

    % --- Kompressionsfaktor F_P ---
    dP = P - P0;
    dP2 = (P.^2 - P0.^2)/2;

    term1 = dP .* (c1 + c2*T + c3*T.^2 + c4*T.^3 + c5*T.^4 + c6*T.^5 + ...
                   S.*(d1 + d2*T + d3*T.^2));
    term2 = dP2 .* (c7 + c8*T + c9*T.^3 + d4*S);

    F_P = exp(term1 + term2);

    % --- Gesamtdichte ---
    rho_sw = rho_0 .* F_P;
end

== matlab function AGMD_model_R2024b/Subsystem/Hot Channel/MATLAB Function ==
  data: T_mittel input; y output; T_h_ein input; cp input; m input; T_h_aus output
function [y ,T_h_aus] = fcn(T_mittel, T_h_ein,cp,m)

% Determination of outgoing temperatures

T_h_aus = T_mittel*2 - T_h_ein;

% Determination of heat flow
y = cp * m * (T_h_ein- T_h_aus);
